simulink model "adaptive_equalization_simulink"  (R2016b)
settings: Solver=VariableStepDiscrete  StartTime=0.0  StopTime=inf  RelTol=1e-3
values from neighbouring files (symbols this model uses):
  coptD = sig2a*inv(PSIy)*conj(gD_)    [MSE_matlab2.m]    (also in adaptive_equalization.m)
  D = posMSED    [MSE_matlab2.m]    (also in adaptive_equalization.m; channel_coding_matlab.m = sum(C,2))
  gk = gk/Kg    [MSE_matlab2.m]    (also in adaptive_equalization.m)
  M = 8    [ML_receiver_matlab.m]    (also in MSE_matlab2.m = 16; OFDM1.m = 64; adaptive_equalization.m = 16)
libraries: dspstat3 x2, commchan3 x1, commrandsrc3 x1, commdigbbndam3 x1, dspbuff3 x1
settings Model: Creator=Shu  LastModifiedBy=Shu
settings DataIOCC: LimitDataPoints=on  SaveOutput=off  SaveTime=off
settings OptimizationCC: BooleanDataType=off  DefaultParameterBehavior=Inlined  LocalBlockOutputs=off  LifeSpan=inf
settings DebuggingCC: AlgebraicLoopMsg=error  SingleTaskRateTransMsg=error  AllowSymbolicDim=off  SFUnexpectedBacktrackingDiag=warning  SFNoUnconditionalDefaultTransitionDiag=warning  SFExecutionAtInitializationDiag=none
settings GRTTargetCC: TargetLangStandard=C89/C90 (ANSI)  GeneratePreprocessorConditionals=Disable all
settings ConfigComp: CovMetricSettings=dw  CovHtmlReporting=on  CovSaveCumulativeToWorkspaceVar=on  CovSaveSingleToWorkspaceVar=on  CovExternalEMLEnable=off  CovSFcnEnable=off

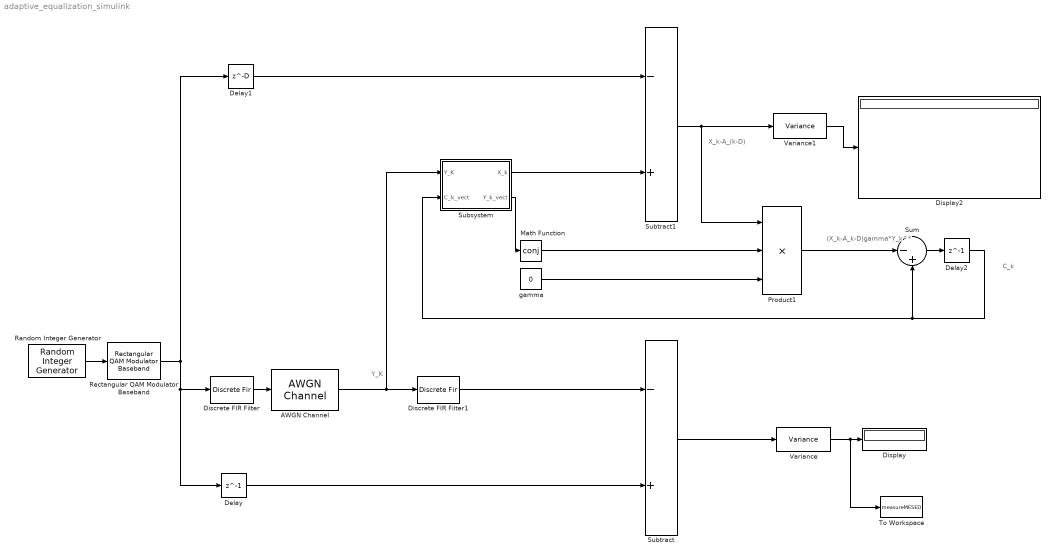
== system adaptive_equalization_simulink ==
  note: Y_K
  note: (X_k-A_k-D)gamma*Y_k^*
  note: C_k
  note: X_k-A_(k-D)
  AWGN Channel : commchan3/AWGN Channel  InputProcessing=Columns as channels (frame based)  seed=67  noiseMode="Signal to noise ratio  (SNR)"  EbNodB=10  EsNodB=10  SNRdB=SNRdB  bitsPerSym=1  Ps=2*(M-1)/3  Tsym=1  variance=1
  Delay : Delay  DelayLength=1  InitialCondition=0
  Delay1 : Delay  DelayLength=D  InitialCondition=0
  Delay2 : Delay  DelayLength=1  InitialCondition=coptD
  Discrete FIR Filter : DiscreteFir  Coefficients=gk  InputProcessing=Columns as channels (frame based)
  Discrete FIR Filter1 : DiscreteFir  Coefficients=coptD.'  InputProcessing=Columns as channels (frame based)
  Display : Display
  Display2 : Display
  Math Function : Math  Operator=conj  SaturateOnIntegerOverflow=on
  Product1 : Product  Inputs=3
  Random Integer Generator : commrandsrc3/Random Integer Generator  SetSize=M  SeedSource=Auto  Seed=0  SampleTime=1  SamplesPerFrame=1  OutputDataType=double  SimulateUsing=Interpreted execution
  Rectangular QAM Modulator Baseband : commdigbbndam3/Rectangular QAM Modulator Baseband  M=M  InType=Integer  Enc=Gray  Mapping=[0:15]  PowType=Min. distance between symbols  MinDist=2  AvgPow=1  PeakPow=1  Ph=0  outDtype=double  outWordLen=16  outUDDataType=sfix(16)  outFracLenMode=Best precision  outFracLen=15  outDataTypeStr=double  outLastDataTypeStr=double
  Subsystem : Subsystem
  Subtract : Sum  Inputs=-+
  Subtract1 : Sum  Inputs=-+
  Sum : Sum  Inputs=|-+
  To Workspace : ToWorkspace  VariableName=measureMESED  SampleTime=-1
      settings: MaxDataPoints=1
  Variance : dspstat3/Variance  run=on  reset_popup=None  directionMode=Each column  dimension=1  roiEnable=off  roiType=Rectangles  roiPortion=Entire ROI  roiOutput=Individual statistics for each ROI  roiFlag=off  roundingMode=Floor  overflowMode=off
  Variance1 : dspstat3/Variance  run=on  reset_popup=None  directionMode=Each column  dimension=1  roiEnable=off  roiType=Rectangles  roiPortion=Entire ROI  roiOutput=Individual statistics for each ROI  roiFlag=off  roundingMode=Floor  overflowMode=off
  "gamma " : Constant  Value=0  SampleTime=-1
  wires:
  Random Integer Generator/1 -> Rectangular QAM Modulator Baseband/1
  Rectangular QAM Modulator Baseband/1 -> Delay/1, Discrete FIR Filter/1, Delay1/1
  Discrete FIR Filter/1 -> AWGN Channel/1
  AWGN Channel/1 -> Subsystem/1("Y_K "), Discrete FIR Filter1/1
  Discrete FIR Filter1/1 -> Subtract/1
  Delay/1 -> Subtract/2
  Subtract/1 -> Variance/1
  Variance/1 -> To Workspace/1, Display/1
  Delay1/1 -> Subtract1/1
  Subtract1/1 -> Product1/1, Variance1/1
  Variance1/1 -> Display2/1
  Math Function/1 -> Product1/2
  "gamma "/1 -> Product1/3
  Subsystem/1(X_k) -> Subtract1/2
  Subsystem/2(Y_k_vect) -> Math Function/1
  Delay2/1 -> Sum/2, Subsystem/2("C_k_vect ")
  Product1/1 -> Sum/1
  Sum/1 -> Delay2/1

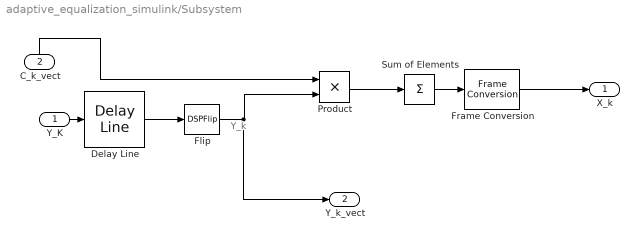
== system adaptive_equalization_simulink/Subsystem ==
  note: Y_k
  "Y_K " : Inport
  "C_k_vect " : Inport  Port=2
  Delay Line : dspbuff3/Delay Line  siz=L  ic=0  directfeed=off  enable_output=off  hold_output=off  TreatMby1Signals=One channel  OutputFrames=off
  Flip : DSPFlip
  Frame Conversion : FrameConversion  InheritSamplingMode=off  OutFrame=Sample-based
  Product : Product
  Sum of Elements : Sum  Inputs=+
  X_k : Outport
  Y_k_vect : Outport  Port=2
  wires:
  Flip/1 -> Y_k_vect/1, Product/2
  Sum of Elements/1 -> Frame Conversion/1
  Delay Line/1 -> Flip/1
  Product/1 -> Sum of Elements/1
  "Y_K "/1 -> Delay Line/1
  "C_k_vect "/1 -> Product/1
  Frame Conversion/1 -> X_k/1
